simulink model "Room32"  (R2016b)
settings: Solver=FixedStepDiscrete  StartTime=0.0  StopTime=100  RelTol=1e-3
settings Model: Creator=3essawy  LastModifiedBy=3essawy
settings OptimizationCC: DefaultParameterBehavior=Inlined
settings DebuggingCC: ParameterTunabilityLossMsg=error
settings RTWCC: SystemTargetFile=ert.tlc  GenCodeOnly=on  TemplateMakefile=ert_default_tmf  Description=Embedded Coder  GenerateReport=on  IncludeHyperlinkInReport=on  LaunchReport=on  GenerateTraceInfo=on  GenerateTraceReport=on  GenerateTraceReportSl=on  GenerateTraceReportSf=on  GenerateTraceReportEml=on
settings CodeAppCC: ForceParamTrailComments=on  IgnoreCustomStorageClasses=off  OperatorAnnotations=on  SimulinkDataObjDesc=on  SFDataObjDesc=on  MATLABFcnDesc=on  InsertBlockDesc=on  MATLABSourceComments=on
settings ERTTargetCC: TargetLangStandard=C99 (ISO)  GenerateSampleERTMain=on  InlinedParameterPlacement=NonHierarchical  ERTCustomFileTemplate=example_file_process.tlc  EnableUserReplacementTypes=on

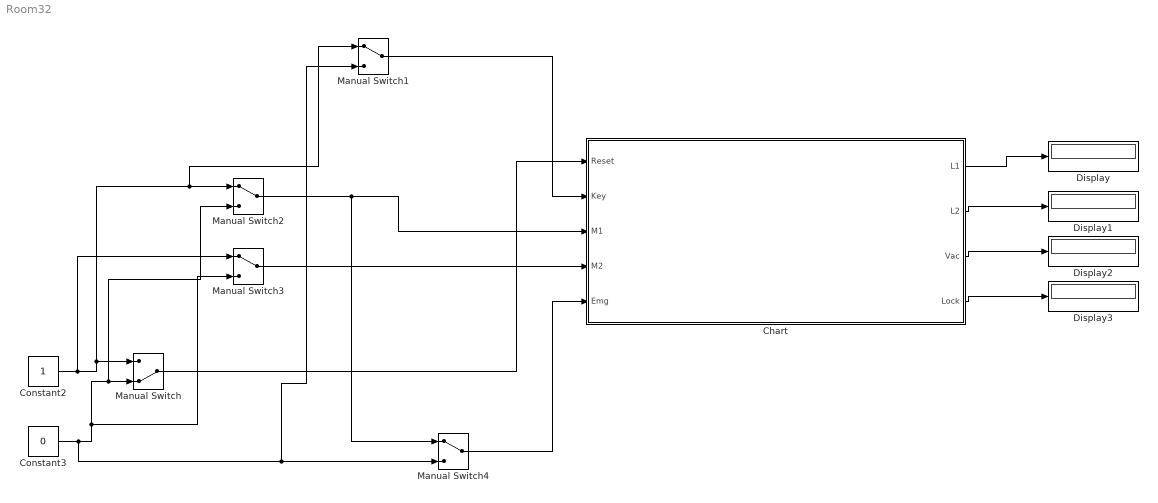
== system Room32 ==
  Chart : Stateflow chart  TreatAsAtomicUnit=on
  Constant2 : Constant
  Constant3 : Constant  Value=0
  Display{,1..3} (4 alike) : Display
  Manual Switch : ManualSwitch  CurrentSetting=0
  Manual Switch{1..4} (4 alike) : ManualSwitch
  wires:
  Chart/1(L1) -> Display/1
  Chart/2(L2) -> Display1/1
  Chart/3(Vac) -> Display2/1
  Chart/4(Lock) -> Display3/1
  Manual Switch/1 -> Chart/1(Reset)
  Constant2/1 -> Manual Switch3/1, Manual Switch1/1, Manual Switch2/1, Manual Switch/1
  Constant3/1 -> Manual Switch1/2, Manual Switch4/2, Manual Switch3/2, Manual Switch2/2, Manual Switch/2
  Manual Switch1/1 -> Chart/2(Key)
  Manual Switch2/1 -> Manual Switch4/1, Chart/3(M1)
  Manual Switch3/1 -> Chart/4(M2)
  Manual Switch4/1 -> Chart/5(Emg)

== stateflow chart Room32/Chart ==
  state Invalid
    entry:
    Lock=1;
    exit:
    Counter=0;
  state R1
    entry:
    L1=1;
    exit:
    L1=0;
  state R2
    entry:
    L2=1;
    exit:
    L2=0;
  state Valid
    entry:
    L1=0;
    L2=0;
  state Vacuum
    entry:
    Vac=1;
    Lock=1;
    exit:
    Vac=0;
    L1=0;
    L2=0;
    exit:
    Counter=0;
  state Emergency
    entry:
    L1=1;
    L2=1;
  (default) -> (junction 7) : {Counter=0;}
  Invalid -> (junction 7) : [Reset==1]
  Vacuum -> (junction 7) : [Reset==1]
  (junction 7) -> (junction 8) [order 1] : [Key==0]
  (junction 7) -> (junction 9) [order 2] : {Counter=0;}
  (junction 8) -> (junction 10) : {Counter = Counter + 1;}
  (junction 10) -> (junction 9)
  (junction 9) -> (junction 11)
  (junction 11) -> (junction 18)
  (junction 18) -> (junction 19) [order 1] : [Counter==3]
  (junction 18) -> (junction 20) [order 2] : {Valid=1;}
  (junction 19) -> (junction 21) : {Valid=0;}
  (junction 21) -> (junction 20) [order 1] : [Valid==1]
  (junction 21) -> Invalid [order 2]
  (junction 20) -> (junction 22)
  (junction 22) -> Valid
  Valid -> R2 [order 2] : [M2==1]
  Valid -> R1 [order 1] : [M1==1]
  R2 -> Valid [order 1] : [M2==0]
  R1 -> Valid [order 1] : [M1==0]
  Valid -> Emergency [order 3] : [Emg==1]
  R2 -> Emergency [order 2] : [Emg==1]
  R1 -> Emergency [order 2] : [Emg==1]
  Emergency -> Vacuum : after(5,sec)
  data: Reset input; Key input; L1 output; L2 output; Vac output; Lock output; Valid local; Counter local; M1 input; M2 input; Emg input
